simulink model "Combined_model"  (R2019b)
settings: Solver=VariableStepAuto  StartTime=0.0  StopTime=15  RelTol=1e-6
undefined symbols (not defined in the file or in its folder): D0, D_e, dD0, dE0, dI0, dJ0, dR0, dS0, E0, I0, J0, R0, R_e, S0, S_e, u_e
settings Model: Creator=felipeareces  LastModifiedBy=felipeareces

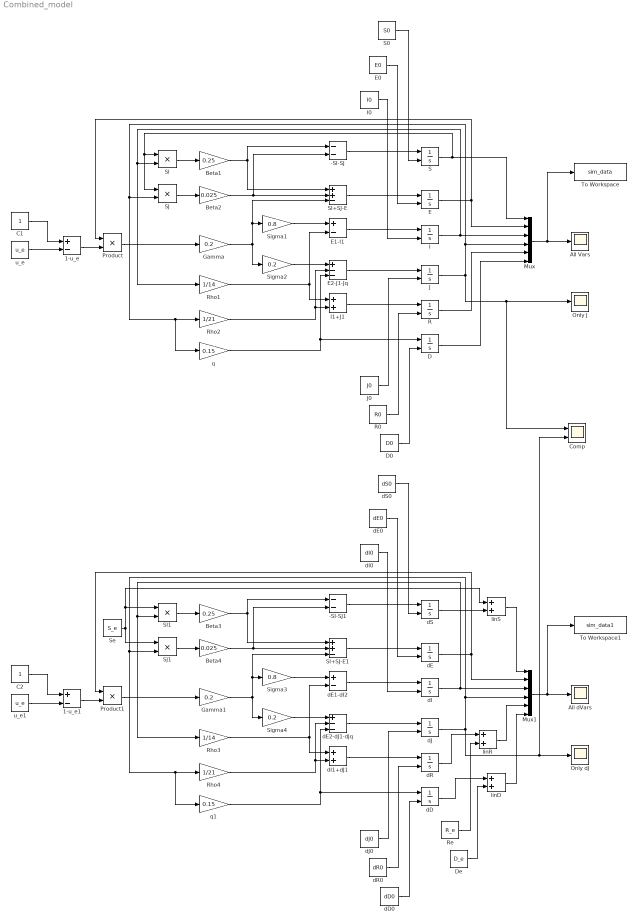
== system Combined_model ==
  -SI-SJ : Sum  Inputs=--
  -SI-SJ1 : Sum  Inputs=--
  1-u_e : Sum  Inputs=+-
  1-u_e1 : Sum  Inputs=+-
  All Vars : Scope
  All dVars : Scope
  Beta1 : Gain  Gain=0.25
  Beta2 : Gain  Gain=0.025
  Beta3 : Gain  Gain=0.25
  Beta4 : Gain  Gain=0.025
  C1 : Constant
  C2 : Constant
  Comp : Scope  NumInputPorts=2
  D : Integrator  InitialConditionSource=external
  D0 : Constant  Value=D0
  De : Constant  Value=D_e
  E : Integrator  InitialConditionSource=external
  E0 : Constant  Value=E0
  E1-I1 : Sum  Inputs=+-
  E2-J1-Jq : Sum  Inputs=+--
  Gamma : Gain  Gain=0.2
  Gamma1 : Gain  Gain=0.2
  I : Integrator  InitialConditionSource=external
  I0 : Constant  Value=I0
  I1+J1 : Sum
  J : Integrator  InitialConditionSource=external
  J0 : Constant  Value=J0
  Mux : Mux  Inputs=6
  Mux1 : Mux  Inputs=6
  Only J : Scope
  Only dJ : Scope
  Product : Product
  Product1 : Product
  R : Integrator  InitialConditionSource=external
  R0 : Constant  Value=R0
  Re : Constant  Value=R_e
  Rho1 : Gain  Gain=1/14
  Rho2 : Gain  Gain=1/21
  Rho3 : Gain  Gain=1/14
  Rho4 : Gain  Gain=1/21
  S : Integrator  InitialConditionSource=external
  S0 : Constant  Value=S0
  SI : Product
  SI+SJ-E : Sum  Inputs=++-
  SI+SJ-E1 : Sum  Inputs=++-
  SI1 : Product
  SJ : Product
  SJ1 : Product
  Se : Constant  Value=S_e
  Sigma1 : Gain  Gain=0.8
  Sigma2 : Gain  Gain=0.2
  Sigma3 : Gain  Gain=0.8
  Sigma4 : Gain  Gain=0.2
  To Workspace : ToWorkspace  VariableName=sim_data  SaveFormat=Timeseries  SampleTime=-1
  To Workspace1 : ToWorkspace  VariableName=sim_data1  SaveFormat=Timeseries  SampleTime=-1
  dD : Integrator  InitialConditionSource=external
  dD0 : Constant  Value=dD0
  dE : Integrator  InitialConditionSource=external
  dE0 : Constant  Value=dE0
  dE1-dI2 : Sum  Inputs=+-
  dE2-dJ1-dJq : Sum  Inputs=+--
  dI : Integrator  InitialConditionSource=external
  dI0 : Constant  Value=dI0
  dI1+dJ1 : Sum
  dJ : Integrator  InitialConditionSource=external
  dJ0 : Constant  Value=dJ0
  dR : Integrator  InitialConditionSource=external
  dR0 : Constant  Value=dR0
  dS : Integrator  InitialConditionSource=external
  dS0 : Constant  Value=dS0
  linD : Sum
  linR : Sum
  linS : Sum
  q : Gain  Gain=0.15
  q1 : Gain  Gain=0.15
  u_e : Constant  Value=u_e
  u_e1 : Constant  Value=u_e
  wires:
  S0/1 -> S/2
  E0/1 -> E/2
  D0/1 -> D/2
  R0/1 -> R/2
  J0/1 -> J/2
  I0/1 -> I/2
  S/1 -> Mux/1, SJ/1, SI/1
  I/1 -> Mux/3, Rho1/1, SI/2
  SI/1 -> Beta1/1
  J/1 -> Comp/1, Only J/1, Mux/4, q/1, Rho2/1, SJ/2
  SJ/1 -> Beta2/1
  -SI-SJ/1 -> S/1
  Beta1/1 -> SI+SJ-E/1, -SI-SJ/1
  Beta2/1 -> -SI-SJ/2, SI+SJ-E/2
  Gamma/1 -> Sigma2/1, SI+SJ-E/3, Sigma1/1
  E/1 -> Product/1, Mux/2
  SI+SJ-E/1 -> E/1
  Sigma1/1 -> E1-I1/1
  E1-I1/1 -> I/1
  Rho1/1 -> E1-I1/2, I1+J1/1
  Sigma2/1 -> E2-J1-Jq/1
  Rho2/1 -> E2-J1-Jq/2, I1+J1/2
  q/1 -> E2-J1-Jq/3, D/1
  R/1 -> Mux/5
  D/1 -> Mux/6
  I1+J1/1 -> R/1
  E2-J1-Jq/1 -> J/1
  Mux/1 -> To Workspace/1, All Vars/1
  u_e/1 -> 1-u_e/2
  C1/1 -> 1-u_e/1
  1-u_e/1 -> Product/2
  Product/1 -> Gamma/1
  u_e1/1 -> 1-u_e1/2
  dE1-dI2/1 -> dI/1
  q1/1 -> dE2-dJ1-dJq/3, dD/1
  Beta3/1 -> SI+SJ-E1/1, -SI-SJ1/1
  C2/1 -> 1-u_e1/1
  dE2-dJ1-dJq/1 -> dJ/1
  1-u_e1/1 -> Product1/2
  dE/1 -> Product1/1, Mux1/2
  Mux1/1 -> To Workspace1/1, All dVars/1
  SI+SJ-E1/1 -> dE/1
  dD0/1 -> dD/2
  Product1/1 -> Gamma1/1
  dR0/1 -> dR/2
  SJ1/1 -> Beta4/1
  dJ0/1 -> dJ/2
  Sigma3/1 -> dE1-dI2/1
  Rho4/1 -> dE2-dJ1-dJq/2, dI1+dJ1/2
  -SI-SJ1/1 -> dS/1
  Rho3/1 -> dE1-dI2/2, dI1+dJ1/1
  Sigma4/1 -> dE2-dJ1-dJq/1
  dI1+dJ1/1 -> dR/1
  dI0/1 -> dI/2
  dS0/1 -> dS/2
  dE0/1 -> dE/2
  Beta4/1 -> -SI-SJ1/2, SI+SJ-E1/2
  SI1/1 -> Beta3/1
  dI/1 -> Mux1/3, Rho3/1, SI1/2
  dJ/1 -> Comp/2, Only dJ/1, Mux1/4, q1/1, Rho4/1, SJ1/2
  Gamma1/1 -> Sigma4/1, SI+SJ-E1/3, Sigma3/1
  Se/1 -> linS/1, SI1/1, SJ1/1
  dS/1 -> linS/2
  linS/1 -> Mux1/1
  De/1 -> linD/2
  Re/1 -> linR/2
  dD/1 -> linD/1
  linD/1 -> Mux1/6
  dR/1 -> linR/1
  linR/1 -> Mux1/5
